simulink model "model1"  (R2024a)
settings: Solver=VariableStepAuto  StartTime=0.0  StopTime=simulation_time  RelTol=1e-3
values from neighbouring files (symbols this model uses):
  dq_0 = zeros(n, 1)    [example.m]
  path = @(t) circle_center + u_circle_plane*radius*cos((t/T) * (2*pi)) + v_circle_plane*radius*sin((t/T) * (2*pi))    [example.m]
  path_ddot = @(t) -u_circle_plane*radius*(2*pi/T)*(2*pi/T)*cos((t/T) * (2*pi)) - v_circle_plane*radius*(2*pi/T)*(2*pi/T)*sin((t/T) * (2*pi))    [example.m]
  path_dot = @(t) -u_circle_plane*radius*(2*pi/T)*sin((t/T) * (2*pi)) + v_circle_plane*radius*(2*pi/T)*cos((t/T) * (2*pi))    [example.m]
  q_0 = randn(n, 1)    [example.m]
  robot_model = importrobot("../robot_model/kuka-lwr-4plus/model1.urdf", 'DataFormat', 'column')    [example.m]
undefined symbols (not defined in the file or in its folder): torque_low_bound, torque_up_bound, X, Y, Z
libraries: sm_lib x74, nesl_utility x8, robotmaniplib x4
(part 2 of 5)

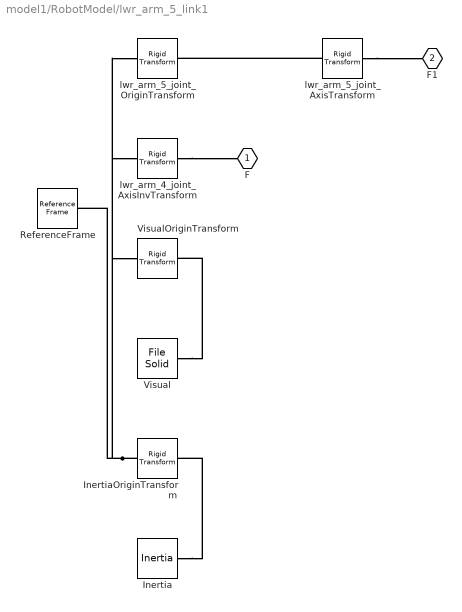
== system model1/RobotModel/lwr_arm_5_link1 ==
  Inertia : sm_lib/Body Elements/Inertia  InertiaType=Custom  Mass=2  MassUnits=kg  CenterOfMass=[0, 0, 0]  CenterOfMassUnits=m  MomentsOfInertia=[0.0126506666667, 0.0108506666667, 0.003]  MomentsOfInertiaUnits=kg*m^2  ProductsOfInertia=[0, 0, 0]  ProductsOfInertiaUnits=kg*m^2  GraphicType=None  MarkerShape=Inertia  MarkerSize=20  GraphicVisPropType=SimpleVisualProperties  GraphicDiffuseColor=[0.5 0.5 0.5]  GraphicOpacity=1  GraphicSpecularColor=[0.5 0.5 0.5 1.0]  GraphicAmbientColor=[0.15 0.15 0.15 1.0]  GraphicEmissiveColor=[0.0 0.0 0.0 1.0]  GraphicShininess=75
  InertiaOriginTransform : sm_lib/Frames and Transforms/Rigid Transform  RotationMethod=RotationSequence  FollAlignAxisA=+X  BaseAlignAxisA=+Y  FollAlignAxisB=+Y  BaseAlignAxisB=+Z  RotationStandardAxis=+Z  RotationAngle=0  RotationAngleUnits=deg  RotationArbitraryAxis=[0 0 1]  RotationSequenceAxes=BaseAxes  RotationSequence=XYZ  RotationSequenceAngles=[0, 0, 0]  RotationSequenceAnglesUnits=rad  RotationMatrix=[1 0 0;0 1 0;0 0 1]  Quaternion=[1 0 0 0]  TranslationMethod=Cartesian  TranslationCartesianOffset=[0, 0, 0.124]  TranslationCartesianOffsetUnits=m  TranslationStandardAxis=+Z  TranslationStandardOffset=0  TranslationStandardOffsetUnits=m  TranslationROffset=0  TranslationROffsetUnits=m  TranslationThetaOffset=0  TranslationThetaOffsetUnits=deg  TranslationZOffset=0  TranslationZOffsetUnits=m
  ReferenceFrame : sm_lib/Frames and Transforms/Reference Frame
  Visual : sm_lib/Body Elements/File Solid  ExtGeomFileName=/Users/salvatore/Desktop/Università/Development/Rob-HW/Damping-in-the-null-space-for-a-redundant-robot/robot_model/kuka-lwr-4plus/meshes/arm_segment_last.stl  UnitType=Custom  ExtGeomFileUnits=m  StepReaderType=HEX  ExportConvexHullGeometry=off  InertiaType=Custom  BasedOnType=DensityFromFile  Density=1000  DensityUnits=kg/m^3  Mass=0  MassUnits=kg  CenterOfMass=[0, 0, 0]  CenterOfMassUnits=m  MomentsOfInertia=[0, 0, 0]  MomentsOfInertiaUnits=kg*m^2  ProductsOfInertia=[0, 0, 0]  ProductsOfInertiaUnits=kg*m^2  GraphicType=FromGeometry  MarkerShape=Sphere  MarkerSize=10  GraphicVisPropType=SimpleVisualProperties  GraphicDiffuseColor=[1, 0.487, 0]  GraphicOpacity=1  GraphicSpecularColor=[0.5 0.5 0.5 1.0]  GraphicAmbientColor=[0.15 0.15 0.15 1.0]  GraphicEmissiveColor=[0.0 0.0 0.0 1.0]  GraphicShininess=75  DoExposeReferenceFrame=on  SerializedFrames=<Frames/>
  VisualOriginTransform : sm_lib/Frames and Transforms/Rigid Transform  RotationMethod=RotationSequence  FollAlignAxisA=+X  BaseAlignAxisA=+Y  FollAlignAxisB=+Y  BaseAlignAxisB=+Z  RotationStandardAxis=+Z  RotationAngle=0  RotationAngleUnits=deg  RotationArbitraryAxis=[0 0 1]  RotationSequenceAxes=BaseAxes  RotationSequence=XYZ  RotationSequenceAngles=[0, 0, -3.141592653589587]  RotationSequenceAnglesUnits=rad  RotationMatrix=[1 0 0;0 1 0;0 0 1]  Quaternion=[1 0 0 0]  TranslationMethod=Cartesian  TranslationCartesianOffset=[0, 0, 0]  TranslationCartesianOffsetUnits=m  TranslationStandardAxis=+Z  TranslationStandardOffset=0  TranslationStandardOffsetUnits=m  TranslationROffset=0  TranslationROffsetUnits=m  TranslationThetaOffset=0  TranslationThetaOffsetUnits=deg  TranslationZOffset=0  TranslationZOffsetUnits=m
  lwr_arm_4_joint_AxisInvTransform : sm_lib/Frames and Transforms/Rigid Transform  RotationMethod=ArbitraryAxis  FollAlignAxisA=+X  BaseAlignAxisA=+Y  FollAlignAxisB=+Y  BaseAlignAxisB=+Z  RotationStandardAxis=+Z  RotationAngle=0  RotationAngleUnits=rad  RotationArbitraryAxis=[1, 0, 0]  RotationSequenceAxes=FollowerAxes  RotationSequence=XYX  RotationSequenceAngles=[0 0 0]  RotationSequenceAnglesUnits=deg  RotationMatrix=[1 0 0;0 1 0;0 0 1]  Quaternion=[1 0 0 0]  TranslationMethod=Cartesian  TranslationCartesianOffset=[0, 0, 0]  TranslationCartesianOffsetUnits=m  TranslationStandardAxis=+Z  TranslationStandardOffset=0  TranslationStandardOffsetUnits=m  TranslationROffset=0  TranslationROffsetUnits=m  TranslationThetaOffset=0  TranslationThetaOffsetUnits=deg  TranslationZOffset=0  TranslationZOffsetUnits=m
  lwr_arm_5_joint_AxisTransform : sm_lib/Frames and Transforms/Rigid Transform  RotationMethod=ArbitraryAxis  FollAlignAxisA=+X  BaseAlignAxisA=+Y  FollAlignAxisB=+Y  BaseAlignAxisB=+Z  RotationStandardAxis=+Z  RotationAngle=1.570796326794897  RotationAngleUnits=rad  RotationArbitraryAxis=[1, 0, 0]  RotationSequenceAxes=FollowerAxes  RotationSequence=XYX  RotationSequenceAngles=[0 0 0]  RotationSequenceAnglesUnits=deg  RotationMatrix=[1 0 0;0 1 0;0 0 1]  Quaternion=[1 0 0 0]  TranslationMethod=Cartesian  TranslationCartesianOffset=[0, 0, 0]  TranslationCartesianOffsetUnits=m  TranslationStandardAxis=+Z  TranslationStandardOffset=0  TranslationStandardOffsetUnits=m  TranslationROffset=0  TranslationROffsetUnits=m  TranslationThetaOffset=0  TranslationThetaOffsetUnits=deg  TranslationZOffset=0  TranslationZOffsetUnits=m
  lwr_arm_5_joint_OriginTransform : sm_lib/Frames and Transforms/Rigid Transform  RotationMethod=RotationSequence  FollAlignAxisA=+X  BaseAlignAxisA=+Y  FollAlignAxisB=+Y  BaseAlignAxisB=+Z  RotationStandardAxis=+Z  RotationAngle=0  RotationAngleUnits=deg  RotationArbitraryAxis=[0 0 1]  RotationSequenceAxes=BaseAxes  RotationSequence=XYZ  RotationSequenceAngles=[0, 0, 0]  RotationSequenceAnglesUnits=rad  RotationMatrix=[1 0 0;0 1 0;0 0 1]  Quaternion=[1 0 0 0]  TranslationMethod=Cartesian  TranslationCartesianOffset=[0, 0, 0.19]  TranslationCartesianOffsetUnits=m  TranslationStandardAxis=+Z  TranslationStandardOffset=0  TranslationStandardOffsetUnits=m  TranslationROffset=0  TranslationROffsetUnits=m  TranslationThetaOffset=0  TranslationThetaOffsetUnits=deg  TranslationZOffset=0  TranslationZOffsetUnits=m
  F : PMIOPort  Side=Left
  F1 : PMIOPort  Port=2  Side=Right
  connections:
  Inertia/RConn1 -- InertiaOriginTransform/RConn1
  InertiaOriginTransform/LConn1 -- ReferenceFrame/RConn1 -- VisualOriginTransform/LConn1 -- lwr_arm_4_joint_AxisInvTransform/LConn1 -- lwr_arm_5_joint_OriginTransform/LConn1
  Visual/RConn1 -- VisualOriginTransform/RConn1
  lwr_arm_4_joint_AxisInvTransform/RConn1 -- F/RConn1
  lwr_arm_5_joint_AxisTransform/RConn1 -- F1/RConn1
  lwr_arm_5_joint_AxisTransform/LConn1 -- lwr_arm_5_joint_OriginTransform/RConn1

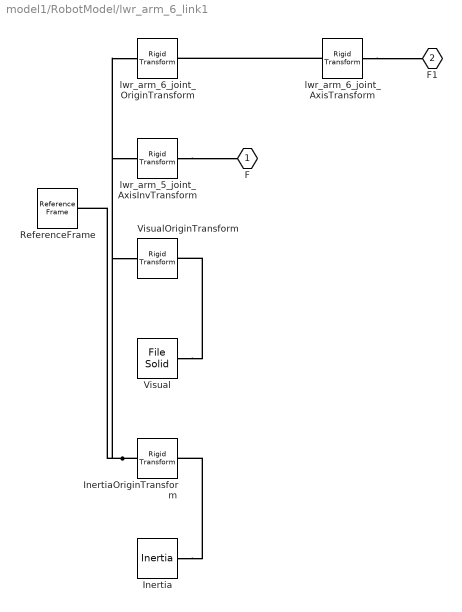
== system model1/RobotModel/lwr_arm_6_link1 ==
  Inertia : sm_lib/Body Elements/Inertia  InertiaType=Custom  Mass=1  MassUnits=kg  CenterOfMass=[0, 0, 0]  CenterOfMassUnits=m  MomentsOfInertia=[0.00260416666667, 0.00260416666667, 0.00260416666667]  MomentsOfInertiaUnits=kg*m^2  ProductsOfInertia=[0, 0, 0]  ProductsOfInertiaUnits=kg*m^2  GraphicType=None  MarkerShape=Inertia  MarkerSize=20  GraphicVisPropType=SimpleVisualProperties  GraphicDiffuseColor=[0.5 0.5 0.5]  GraphicOpacity=1  GraphicSpecularColor=[0.5 0.5 0.5 1.0]  GraphicAmbientColor=[0.15 0.15 0.15 1.0]  GraphicEmissiveColor=[0.0 0.0 0.0 1.0]  GraphicShininess=75
  InertiaOriginTransform : sm_lib/Frames and Transforms/Rigid Transform  RotationMethod=RotationSequence  FollAlignAxisA=+X  BaseAlignAxisA=+Y  FollAlignAxisB=+Y  BaseAlignAxisB=+Z  RotationStandardAxis=+Z  RotationAngle=0  RotationAngleUnits=deg  RotationArbitraryAxis=[0 0 1]  RotationSequenceAxes=BaseAxes  RotationSequence=XYZ  RotationSequenceAngles=[0, 0, 0]  RotationSequenceAnglesUnits=rad  RotationMatrix=[1 0 0;0 1 0;0 0 1]  Quaternion=[1 0 0 0]  TranslationMethod=Cartesian  TranslationCartesianOffset=[0, 0, 0]  TranslationCartesianOffsetUnits=m  TranslationStandardAxis=+Z  TranslationStandardOffset=0  TranslationStandardOffsetUnits=m  TranslationROffset=0  TranslationROffsetUnits=m  TranslationThetaOffset=0  TranslationThetaOffsetUnits=deg  TranslationZOffset=0  TranslationZOffsetUnits=m
  ReferenceFrame : sm_lib/Frames and Transforms/Reference Frame
  Visual : sm_lib/Body Elements/File Solid  ExtGeomFileName=/Users/salvatore/Desktop/Università/Development/Rob-HW/Damping-in-the-null-space-for-a-redundant-robot/robot_model/kuka-lwr-4plus/meshes/arm_wrist.stl  UnitType=Custom  ExtGeomFileUnits=m  StepReaderType=HEX  ExportConvexHullGeometry=off  InertiaType=Custom  BasedOnType=DensityFromFile  Density=1000  DensityUnits=kg/m^3  Mass=0  MassUnits=kg  CenterOfMass=[0, 0, 0]  CenterOfMassUnits=m  MomentsOfInertia=[0, 0, 0]  MomentsOfInertiaUnits=kg*m^2  ProductsOfInertia=[0, 0, 0]  ProductsOfInertiaUnits=kg*m^2  GraphicType=FromGeometry  MarkerShape=Sphere  MarkerSize=10  GraphicVisPropType=SimpleVisualProperties  GraphicDiffuseColor=[0.7, 0.7, 0.7]  GraphicOpacity=1  GraphicSpecularColor=[0.5 0.5 0.5 1.0]  GraphicAmbientColor=[0.15 0.15 0.15 1.0]  GraphicEmissiveColor=[0.0 0.0 0.0 1.0]  GraphicShininess=75  DoExposeReferenceFrame=on  SerializedFrames=<Frames/>
  VisualOriginTransform : sm_lib/Frames and Transforms/Rigid Transform  RotationMethod=RotationSequence  FollAlignAxisA=+X  BaseAlignAxisA=+Y  FollAlignAxisB=+Y  BaseAlignAxisB=+Z  RotationStandardAxis=+Z  RotationAngle=0  RotationAngleUnits=deg  RotationArbitraryAxis=[0 0 1]  RotationSequenceAxes=BaseAxes  RotationSequence=XYZ  RotationSequenceAngles=[0, 0, -3.141592653589587]  RotationSequenceAnglesUnits=rad  RotationMatrix=[1 0 0;0 1 0;0 0 1]  Quaternion=[1 0 0 0]  TranslationMethod=Cartesian  TranslationCartesianOffset=[0, 0, 0]  TranslationCartesianOffsetUnits=m  TranslationStandardAxis=+Z  TranslationStandardOffset=0  TranslationStandardOffsetUnits=m  TranslationROffset=0  TranslationROffsetUnits=m  TranslationThetaOffset=0  TranslationThetaOffsetUnits=deg  TranslationZOffset=0  TranslationZOffsetUnits=m
  lwr_arm_5_joint_AxisInvTransform : sm_lib/Frames and Transforms/Rigid Transform  RotationMethod=ArbitraryAxis  FollAlignAxisA=+X  BaseAlignAxisA=+Y  FollAlignAxisB=+Y  BaseAlignAxisB=+Z  RotationStandardAxis=+Z  RotationAngle=1.570796326794897  RotationAngleUnits=rad  RotationArbitraryAxis=[1, 0, 0]  RotationSequenceAxes=FollowerAxes  RotationSequence=XYX  RotationSequenceAngles=[0 0 0]  RotationSequenceAnglesUnits=deg  RotationMatrix=[1 0 0;0 1 0;0 0 1]  Quaternion=[1 0 0 0]  TranslationMethod=Cartesian  TranslationCartesianOffset=[0, 0, 0]  TranslationCartesianOffsetUnits=m  TranslationStandardAxis=+Z  TranslationStandardOffset=0  TranslationStandardOffsetUnits=m  TranslationROffset=0  TranslationROffsetUnits=m  TranslationThetaOffset=0  TranslationThetaOffsetUnits=deg  TranslationZOffset=0  TranslationZOffsetUnits=m
  lwr_arm_6_joint_AxisTransform : sm_lib/Frames and Transforms/Rigid Transform  RotationMethod=ArbitraryAxis  FollAlignAxisA=+X  BaseAlignAxisA=+Y  FollAlignAxisB=+Y  BaseAlignAxisB=+Z  RotationStandardAxis=+Z  RotationAngle=0  RotationAngleUnits=rad  RotationArbitraryAxis=[1, 0, 0]  RotationSequenceAxes=FollowerAxes  RotationSequence=XYX  RotationSequenceAngles=[0 0 0]  RotationSequenceAnglesUnits=deg  RotationMatrix=[1 0 0;0 1 0;0 0 1]  Quaternion=[1 0 0 0]  TranslationMethod=Cartesian  TranslationCartesianOffset=[0, 0, 0]  TranslationCartesianOffsetUnits=m  TranslationStandardAxis=+Z  TranslationStandardOffset=0  TranslationStandardOffsetUnits=m  TranslationROffset=0  TranslationROffsetUnits=m  TranslationThetaOffset=0  TranslationThetaOffsetUnits=deg  TranslationZOffset=0  TranslationZOffsetUnits=m
  lwr_arm_6_joint_OriginTransform : sm_lib/Frames and Transforms/Rigid Transform  RotationMethod=RotationSequence  FollAlignAxisA=+X  BaseAlignAxisA=+Y  FollAlignAxisB=+Y  BaseAlignAxisB=+Z  RotationStandardAxis=+Z  RotationAngle=0  RotationAngleUnits=deg  RotationArbitraryAxis=[0 0 1]  RotationSequenceAxes=BaseAxes  RotationSequence=XYZ  RotationSequenceAngles=[0, -0, 0]  RotationSequenceAnglesUnits=rad  RotationMatrix=[1 0 0;0 1 0;0 0 1]  Quaternion=[1 0 0 0]  TranslationMethod=Cartesian  TranslationCartesianOffset=[0, 0, 0]  TranslationCartesianOffsetUnits=m  TranslationStandardAxis=+Z  TranslationStandardOffset=0  TranslationStandardOffsetUnits=m  TranslationROffset=0  TranslationROffsetUnits=m  TranslationThetaOffset=0  TranslationThetaOffsetUnits=deg  TranslationZOffset=0  TranslationZOffsetUnits=m
  F : PMIOPort  Side=Left
  F1 : PMIOPort  Port=2  Side=Right
  connections:
  Inertia/RConn1 -- InertiaOriginTransform/RConn1
  InertiaOriginTransform/LConn1 -- ReferenceFrame/RConn1 -- VisualOriginTransform/LConn1 -- lwr_arm_5_joint_AxisInvTransform/LConn1 -- lwr_arm_6_joint_OriginTransform/LConn1
  Visual/RConn1 -- VisualOriginTransform/RConn1
  lwr_arm_5_joint_AxisInvTransform/RConn1 -- F/RConn1
  lwr_arm_6_joint_AxisTransform/RConn1 -- F1/RConn1
  lwr_arm_6_joint_AxisTransform/LConn1 -- lwr_arm_6_joint_OriginTransform/RConn1

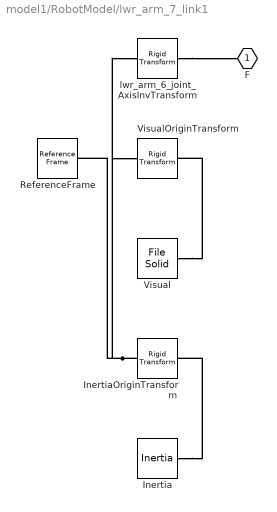
== system model1/RobotModel/lwr_arm_7_link1 ==
  Inertia : sm_lib/Body Elements/Inertia  InertiaType=Custom  Mass=0.2  MassUnits=kg  CenterOfMass=[0, 0, 0]  CenterOfMassUnits=m  MomentsOfInertia=[6.66666666667e-05, 6.66666666667e-05, 0.00012]  MomentsOfInertiaUnits=kg*m^2  ProductsOfInertia=[0, 0, 0]  ProductsOfInertiaUnits=kg*m^2  GraphicType=None  MarkerShape=Inertia  MarkerSize=20  GraphicVisPropType=SimpleVisualProperties  GraphicDiffuseColor=[0.5 0.5 0.5]  GraphicOpacity=1  GraphicSpecularColor=[0.5 0.5 0.5 1.0]  GraphicAmbientColor=[0.15 0.15 0.15 1.0]  GraphicEmissiveColor=[0.0 0.0 0.0 1.0]  GraphicShininess=75
  InertiaOriginTransform : sm_lib/Frames and Transforms/Rigid Transform  RotationMethod=RotationSequence  FollAlignAxisA=+X  BaseAlignAxisA=+Y  FollAlignAxisB=+Y  BaseAlignAxisB=+Z  RotationStandardAxis=+Z  RotationAngle=0  RotationAngleUnits=deg  RotationArbitraryAxis=[0 0 1]  RotationSequenceAxes=BaseAxes  RotationSequence=XYZ  RotationSequenceAngles=[0, 0, 0]  RotationSequenceAnglesUnits=rad  RotationMatrix=[1 0 0;0 1 0;0 0 1]  Quaternion=[1 0 0 0]  TranslationMethod=Cartesian  TranslationCartesianOffset=[0, 0, 0]  TranslationCartesianOffsetUnits=m  TranslationStandardAxis=+Z  TranslationStandardOffset=0  TranslationStandardOffsetUnits=m  TranslationROffset=0  TranslationROffsetUnits=m  TranslationThetaOffset=0  TranslationThetaOffsetUnits=deg  TranslationZOffset=0  TranslationZOffsetUnits=m
  ReferenceFrame : sm_lib/Frames and Transforms/Reference Frame
  Visual : sm_lib/Body Elements/File Solid  ExtGeomFileName=/Users/salvatore/Desktop/Università/Development/Rob-HW/Damping-in-the-null-space-for-a-redundant-robot/robot_model/kuka-lwr-4plus/meshes/arm_flanche.stl  UnitType=Custom  ExtGeomFileUnits=m  StepReaderType=HEX  ExportConvexHullGeometry=off  InertiaType=Custom  BasedOnType=DensityFromFile  Density=1000  DensityUnits=kg/m^3  Mass=0  MassUnits=kg  CenterOfMass=[0, 0, 0]  CenterOfMassUnits=m  MomentsOfInertia=[0, 0, 0]  MomentsOfInertiaUnits=kg*m^2  ProductsOfInertia=[0, 0, 0]  ProductsOfInertiaUnits=kg*m^2  GraphicType=FromGeometry  MarkerShape=Sphere  MarkerSize=10  GraphicVisPropType=SimpleVisualProperties  GraphicDiffuseColor=[0.7, 0.7, 0.7]  GraphicOpacity=1  GraphicSpecularColor=[0.5 0.5 0.5 1.0]  GraphicAmbientColor=[0.15 0.15 0.15 1.0]  GraphicEmissiveColor=[0.0 0.0 0.0 1.0]  GraphicShininess=75  DoExposeReferenceFrame=on  SerializedFrames=<Frames/>
  VisualOriginTransform : sm_lib/Frames and Transforms/Rigid Transform  RotationMethod=RotationSequence  FollAlignAxisA=+X  BaseAlignAxisA=+Y  FollAlignAxisB=+Y  BaseAlignAxisB=+Z  RotationStandardAxis=+Z  RotationAngle=0  RotationAngleUnits=deg  RotationArbitraryAxis=[0 0 1]  RotationSequenceAxes=BaseAxes  RotationSequence=XYZ  RotationSequenceAngles=[0, 0, 0]  RotationSequenceAnglesUnits=rad  RotationMatrix=[1 0 0;0 1 0;0 0 1]  Quaternion=[1 0 0 0]  TranslationMethod=Cartesian  TranslationCartesianOffset=[0, 0, 0]  TranslationCartesianOffsetUnits=m  TranslationStandardAxis=+Z  TranslationStandardOffset=0  TranslationStandardOffsetUnits=m  TranslationROffset=0  TranslationROffsetUnits=m  TranslationThetaOffset=0  TranslationThetaOffsetUnits=deg  TranslationZOffset=0  TranslationZOffsetUnits=m
  lwr_arm_6_joint_AxisInvTransform : sm_lib/Frames and Transforms/Rigid Transform  RotationMethod=ArbitraryAxis  FollAlignAxisA=+X  BaseAlignAxisA=+Y  FollAlignAxisB=+Y  BaseAlignAxisB=+Z  RotationStandardAxis=+Z  RotationAngle=0  RotationAngleUnits=rad  RotationArbitraryAxis=[1, 0, 0]  RotationSequenceAxes=FollowerAxes  RotationSequence=XYX  RotationSequenceAngles=[0 0 0]  RotationSequenceAnglesUnits=deg  RotationMatrix=[1 0 0;0 1 0;0 0 1]  Quaternion=[1 0 0 0]  TranslationMethod=Cartesian  TranslationCartesianOffset=[0, 0, 0]  TranslationCartesianOffsetUnits=m  TranslationStandardAxis=+Z  TranslationStandardOffset=0  TranslationStandardOffsetUnits=m  TranslationROffset=0  TranslationROffsetUnits=m  TranslationThetaOffset=0  TranslationThetaOffsetUnits=deg  TranslationZOffset=0  TranslationZOffsetUnits=m
  F : PMIOPort  Side=Left
  connections:
  Inertia/RConn1 -- InertiaOriginTransform/RConn1
  InertiaOriginTransform/LConn1 -- ReferenceFrame/RConn1 -- VisualOriginTransform/LConn1 -- lwr_arm_6_joint_AxisInvTransform/LConn1
  Visual/RConn1 -- VisualOriginTransform/RConn1
  lwr_arm_6_joint_AxisInvTransform/RConn1 -- F/RConn1

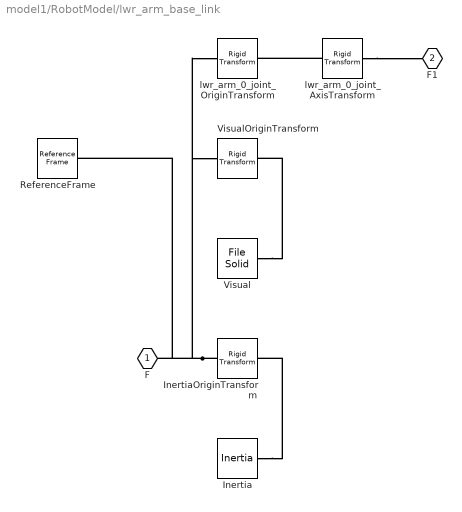
== system model1/RobotModel/lwr_arm_base_link ==
  Inertia : sm_lib/Body Elements/Inertia  InertiaType=Custom  Mass=1.2  MassUnits=kg  CenterOfMass=[0, 0, 0]  CenterOfMassUnits=m  MomentsOfInertia=[0.00229, 0.00216, 0.00229]  MomentsOfInertiaUnits=kg*m^2  ProductsOfInertia=[0, 0, 0]  ProductsOfInertiaUnits=kg*m^2  GraphicType=None  MarkerShape=Inertia  MarkerSize=20  GraphicVisPropType=SimpleVisualProperties  GraphicDiffuseColor=[0.5 0.5 0.5]  GraphicOpacity=1  GraphicSpecularColor=[0.5 0.5 0.5 1.0]  GraphicAmbientColor=[0.15 0.15 0.15 1.0]  GraphicEmissiveColor=[0.0 0.0 0.0 1.0]  GraphicShininess=75
  InertiaOriginTransform : sm_lib/Frames and Transforms/Rigid Transform  RotationMethod=RotationSequence  FollAlignAxisA=+X  BaseAlignAxisA=+Y  FollAlignAxisB=+Y  BaseAlignAxisB=+Z  RotationStandardAxis=+Z  RotationAngle=0  RotationAngleUnits=deg  RotationArbitraryAxis=[0 0 1]  RotationSequenceAxes=BaseAxes  RotationSequence=XYZ  RotationSequenceAngles=[0, 0, 0]  RotationSequenceAnglesUnits=rad  RotationMatrix=[1 0 0;0 1 0;0 0 1]  Quaternion=[1 0 0 0]  TranslationMethod=Cartesian  TranslationCartesianOffset=[0, 0, 0.055]  TranslationCartesianOffsetUnits=m  TranslationStandardAxis=+Z  TranslationStandardOffset=0  TranslationStandardOffsetUnits=m  TranslationROffset=0  TranslationROffsetUnits=m  TranslationThetaOffset=0  TranslationThetaOffsetUnits=deg  TranslationZOffset=0  TranslationZOffsetUnits=m
  ReferenceFrame : sm_lib/Frames and Transforms/Reference Frame
  Visual : sm_lib/Body Elements/File Solid  ExtGeomFileName=/Users/salvatore/Desktop/Università/Development/Rob-HW/Damping-in-the-null-space-for-a-redundant-robot/robot_model/kuka-lwr-4plus/meshes/arm_base.stl  UnitType=Custom  ExtGeomFileUnits=m  StepReaderType=HEX  ExportConvexHullGeometry=off  InertiaType=Custom  BasedOnType=DensityFromFile  Density=1000  DensityUnits=kg/m^3  Mass=0  MassUnits=kg  CenterOfMass=[0, 0, 0]  CenterOfMassUnits=m  MomentsOfInertia=[0, 0, 0]  MomentsOfInertiaUnits=kg*m^2  ProductsOfInertia=[0, 0, 0]  ProductsOfInertiaUnits=kg*m^2  GraphicType=FromGeometry  MarkerShape=Sphere  MarkerSize=10  GraphicVisPropType=SimpleVisualProperties  GraphicDiffuseColor=[1, 0.487, 0]  GraphicOpacity=1  GraphicSpecularColor=[0.5 0.5 0.5 1.0]  GraphicAmbientColor=[0.15 0.15 0.15 1.0]  GraphicEmissiveColor=[0.0 0.0 0.0 1.0]  GraphicShininess=75  DoExposeReferenceFrame=on  SerializedFrames=<Frames/>
  VisualOriginTransform : sm_lib/Frames and Transforms/Rigid Transform  RotationMethod=RotationSequence  FollAlignAxisA=+X  BaseAlignAxisA=+Y  FollAlignAxisB=+Y  BaseAlignAxisB=+Z  RotationStandardAxis=+Z  RotationAngle=0  RotationAngleUnits=deg  RotationArbitraryAxis=[0 0 1]  RotationSequenceAxes=BaseAxes  RotationSequence=XYZ  RotationSequenceAngles=[0, 0, 0]  RotationSequenceAnglesUnits=rad  RotationMatrix=[1 0 0;0 1 0;0 0 1]  Quaternion=[1 0 0 0]  TranslationMethod=Cartesian  TranslationCartesianOffset=[0, 0, 0]  TranslationCartesianOffsetUnits=m  TranslationStandardAxis=+Z  TranslationStandardOffset=0  TranslationStandardOffsetUnits=m  TranslationROffset=0  TranslationROffsetUnits=m  TranslationThetaOffset=0  TranslationThetaOffsetUnits=deg  TranslationZOffset=0  TranslationZOffsetUnits=m
  lwr_arm_0_joint_AxisTransform : sm_lib/Frames and Transforms/Rigid Transform  RotationMethod=ArbitraryAxis  FollAlignAxisA=+X  BaseAlignAxisA=+Y  FollAlignAxisB=+Y  BaseAlignAxisB=+Z  RotationStandardAxis=+Z  RotationAngle=0  RotationAngleUnits=rad  RotationArbitraryAxis=[1, 0, 0]  RotationSequenceAxes=FollowerAxes  RotationSequence=XYX  RotationSequenceAngles=[0 0 0]  RotationSequenceAnglesUnits=deg  RotationMatrix=[1 0 0;0 1 0;0 0 1]  Quaternion=[1 0 0 0]  TranslationMethod=Cartesian  TranslationCartesianOffset=[0, 0, 0]  TranslationCartesianOffsetUnits=m  TranslationStandardAxis=+Z  TranslationStandardOffset=0  TranslationStandardOffsetUnits=m  TranslationROffset=0  TranslationROffsetUnits=m  TranslationThetaOffset=0  TranslationThetaOffsetUnits=deg  TranslationZOffset=0  TranslationZOffsetUnits=m
  lwr_arm_0_joint_OriginTransform : sm_lib/Frames and Transforms/Rigid Transform  RotationMethod=RotationSequence  FollAlignAxisA=+X  BaseAlignAxisA=+Y  FollAlignAxisB=+Y  BaseAlignAxisB=+Z  RotationStandardAxis=+Z  RotationAngle=0  RotationAngleUnits=deg  RotationArbitraryAxis=[0 0 1]  RotationSequenceAxes=BaseAxes  RotationSequence=XYZ  RotationSequenceAngles=[0, 0, 0]  RotationSequenceAnglesUnits=rad  RotationMatrix=[1 0 0;0 1 0;0 0 1]  Quaternion=[1 0 0 0]  TranslationMethod=Cartesian  TranslationCartesianOffset=[0, 0, 0.11]  TranslationCartesianOffsetUnits=m  TranslationStandardAxis=+Z  TranslationStandardOffset=0  TranslationStandardOffsetUnits=m  TranslationROffset=0  TranslationROffsetUnits=m  TranslationThetaOffset=0  TranslationThetaOffsetUnits=deg  TranslationZOffset=0  TranslationZOffsetUnits=m
  F : PMIOPort  Side=Left
  F1 : PMIOPort  Port=2  Side=Right
  connections:
  Inertia/RConn1 -- InertiaOriginTransform/RConn1
  ReferenceFrame/RConn1 -- InertiaOriginTransform/LConn1 -- VisualOriginTransform/LConn1 -- lwr_arm_0_joint_OriginTransform/LConn1 -- F/RConn1
  Visual/RConn1 -- VisualOriginTransform/RConn1
  lwr_arm_0_joint_AxisTransform/RConn1 -- F1/RConn1
  lwr_arm_0_joint_AxisTransform/LConn1 -- lwr_arm_0_joint_OriginTransform/RConn1

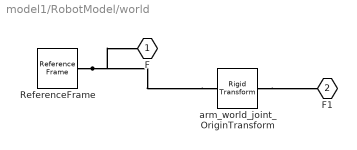
== system model1/RobotModel/world ==
  ReferenceFrame : sm_lib/Frames and Transforms/Reference Frame
  arm_world_joint_OriginTransform : sm_lib/Frames and Transforms/Rigid Transform  RotationMethod=RotationSequence  FollAlignAxisA=+X  BaseAlignAxisA=+Y  FollAlignAxisB=+Y  BaseAlignAxisB=+Z  RotationStandardAxis=+Z  RotationAngle=0  RotationAngleUnits=deg  RotationArbitraryAxis=[0 0 1]  RotationSequenceAxes=BaseAxes  RotationSequence=XYZ  RotationSequenceAngles=[0, 0, 0]  RotationSequenceAnglesUnits=rad  RotationMatrix=[1 0 0;0 1 0;0 0 1]  Quaternion=[1 0 0 0]  TranslationMethod=Cartesian  TranslationCartesianOffset=[0, 0, 0.01]  TranslationCartesianOffsetUnits=m  TranslationStandardAxis=+Z  TranslationStandardOffset=0  TranslationStandardOffsetUnits=m  TranslationROffset=0  TranslationROffsetUnits=m  TranslationThetaOffset=0  TranslationThetaOffsetUnits=deg  TranslationZOffset=0  TranslationZOffsetUnits=m
  F : PMIOPort  Side=Left
  F1 : PMIOPort  Port=2  Side=Right
  connections:
  arm_world_joint_OriginTransform/LConn1 -- ReferenceFrame/RConn1 -- F/RConn1
  arm_world_joint_OriginTransform/RConn1 -- F1/RConn1

== matlab function model1/MATLAB Function ==
  data: configuration input; g_num output
function g_num = g_num(configuration)
%G_NUM1
%    G_NUM = G_NUM1(Q1,Q2,Q3,Q4,Q5)

%    This function was generated by the Symbolic Math Toolbox version 24.1.
%    01-Jul-2024 12:17:42

q1 = configuration(1);
q2 = configuration(2);
q3 = configuration(3);
q4 = configuration(4);
q5 = configuration(5);

t2 = cos(q1);
t3 = cos(q2);
t4 = cos(q3);
t5 = cos(q4);
t6 = cos(q5);
t7 = sin(q1);
t8 = sin(q2);
t9 = sin(q3);
t10 = sin(q4);
t11 = sin(q5);
t12 = t2.*t4;
t13 = t2.*t9;
t14 = t3.*t4.*t7;
t15 = t3.*t7.*t9;
t16 = -t15;
t17 = t13+t14;
t18 = t12+t16;
mt1 = [t7.*(9.31e+2./2.5e+2)-t2.*t8.*3.0772e+1-t4.*t7.*(9.31e+2./2.5e+2)-t3.*t13.*(9.31e+2./2.5e+2)-t2.*t5.*t8.*1.36024e+1+t4.*t6.*t7.*2.4304+t3.*t6.*t13.*2.4304+t3.*t10.*t12.*1.36024e+1-t7.*t9.*t10.*1.36024e+1+t2.*t8.*t10.*t11.*2.4304+t3.*t5.*t11.*t12.*2.4304-t5.*t7.*t9.*t11.*2.4304];
mt2 = [t7.*(t3.*3.14e+2+t3.*t5.*(6.94e+2./5.0)-t8.*t9.*3.8e+1+t4.*t8.*t10.*(6.94e+2./5.0)+t6.*t8.*t9.*(1.24e+2./5.0)-t3.*t10.*t11.*(1.24e+2./5.0)+t4.*t5.*t8.*t11.*(1.24e+2./5.0)).*(-4.9e+1./5.0e+2);t13.*(-9.31e+2./2.5e+2)-t14.*(9.31e+2./2.5e+2)+t6.*t17.*2.4304+t10.*t18.*1.36024e+1+t5.*t11.*t18.*2.4304;t11.*(t10.*t17-t5.*t7.*t8).*(-2.4304)+t5.*t17.*1.36024e+1+t7.*t8.*t10.*1.36024e+1];
mt3 = [t6.*(t5.*t17+t7.*t8.*t10).*2.4304+t11.*t18.*2.4304;0.0;0.0];
g_num = [mt1;mt2;mt3];
end

== matlab function model1/Feeback linearization acceleration ==
  data: f_q input; tau output; dq input; p_d input; dp_d input; ddp_d input; j input; g_q input; c input; M input; jdot input
function tau = FBLAcceleration(f_q, dq, p_d, dp_d, ddp_d, j, g_q, c, M, jdot)

% Control gains
K_P = 100;
K_D = 10;

K_V = 10;
K_M = 10;

% Acceleration command of the FBL controller
% a   = ddq_d + K_P*(q_d - q) + K_D*(dq_d - dq);

% tau = j' * K_P * (p_d - f_q) + K_D * (pinv(j)*dp_d - dq) + g_q;
% end

Winv = M; % the inverse of the weight matrix: can be inverse of eye(7), m^-1, m^-2 
% F = j * pinv(M);
% Finv = pinv(F);
F = j / M; % equivalent to j * inv(M)
Finv = (Winv * F') / (F * Winv * F'); % the weighted pseudo-inverse of F = W^-1*F'*(F*W^-1*F')^-1
a = ddp_d + K_D*(dp_d - j*dq) + K_P*(p_d - f_q);
u0 = zeros(7,1);  % No null space term / no damping
% u0 = -K_V * dq;  % velocity damping
% u0 = -K_M * M * dq;  % momentum damping
tau = Finv * (a - jdot*dq + F*(c + g_q)) + (eye(7) - Finv*F)*u0;

end

== matlab function model1/MATLAB Function1 ==
  data: configuration input; j output
function j = analytic_jacobian(configuration)
%ANALYTIC_JACOBIAN1
%    J = ANALYTIC_JACOBIAN1(Q1,Q2,Q3,Q4)

%    This function was generated by the Symbolic Math Toolbox version 24.1.
%    02-Jul-2024 11:08:16

q1 = configuration(1);
q2 = configuration(2);
q3 = configuration(3);
q4 = configuration(4);

t2 = cos(q1);
t3 = cos(q2);
t4 = cos(q3);
t5 = cos(q4);
t6 = sin(q1);
t7 = sin(q2);
t8 = sin(q3);
t9 = sin(q4);
t10 = t2.*t8;
t11 = t6.*t8;
t12 = t2.*t3.*t4;
t13 = t3.*t4.*t6;
t14 = -t12;
t15 = t10+t13;
t16 = t11+t14;
mt1 = [t6.*t7.*(2.0./5.0)-t9.*t15.*(3.9e+1./1.0e+2)+t5.*t6.*t7.*(3.9e+1./1.0e+2),t2.*t7.*(-2.0./5.0)-t9.*t16.*(3.9e+1./1.0e+2)-t2.*t5.*t7.*(3.9e+1./1.0e+2),0.0,t2.*t3.*(-2.0./5.0)-t2.*t3.*t5.*(3.9e+1./1.0e+2)-t2.*t4.*t7.*t9.*(3.9e+1./1.0e+2),t3.*t6.*(-2.0./5.0)-t3.*t5.*t6.*(3.9e+1./1.0e+2)-t4.*t6.*t7.*t9.*(3.9e+1./1.0e+2),t7.*(-2.0./5.0)-t5.*t7.*(3.9e+1./1.0e+2)+t3.*t4.*t9.*(3.9e+1./1.0e+2),t9.*(t4.*t6+t3.*t10).*(-3.9e+1./1.0e+2),t9.*(t2.*t4-t3.*t11).*(3.9e+1./1.0e+2),t7.*t8.*t9.*(-3.9e+1./1.0e+2)];
mt2 = [t5.*t16.*(-3.9e+1./1.0e+2)+t2.*t7.*t9.*(3.9e+1./1.0e+2),t5.*t15.*(3.9e+1./1.0e+2)+t6.*t7.*t9.*(3.9e+1./1.0e+2),t3.*t9.*(-3.9e+1./1.0e+2)+t4.*t5.*t7.*(3.9e+1./1.0e+2),0.0,0.0,0.0,0.0,0.0,0.0,0.0,0.0,0.0];
j = reshape([mt1,mt2],3,7);
end

== matlab function model1/MATLAB Function3 ==
  data: currJointPos input; j_dot output; currJointVel input
function j_dot = analytic_j_dot1(currJointPos, currJointVel)
%ANALYTIC_J_DOT1
%    J_DOT = ANALYTIC_J_DOT1(Q1,Q2,Q3,Q4,Q_DOT1,Q_DOT2,Q_DOT3,Q_DOT4)

%    This function was generated by the Symbolic Math Toolbox version 24.1.
%    02-Jul-2024 11:08:30

q1 = currJointPos(1);
q_dot1 = currJointVel(1);
q2 = currJointPos(2);
q_dot2 = currJointVel(2);
q3 = currJointPos(3);
q_dot3 = currJointVel(3);
q4 = currJointPos(4);
q_dot4 = currJointVel(4);

t2 = cos(q1);
t3 = cos(q2);
t4 = cos(q3);
t5 = cos(q4);
t6 = sin(q1);
t7 = sin(q2);
t8 = sin(q3);
t9 = sin(q4);
t10 = t2.*t8;
t11 = t6.*t8;
t12 = q_dot3.*t2.*t4;
t14 = q_dot3.*t4.*t6;
t16 = t2.*t3.*t4;
t17 = t3.*t4.*t6;
t20 = q_dot2.*t2.*t4.*t7;
t22 = q_dot2.*t4.*t6.*t7;
t13 = q_dot1.*t10;
t15 = q_dot1.*t11;
t18 = q_dot1.*t16;
t19 = q_dot1.*t17;
t21 = q_dot3.*t3.*t10;
t23 = q_dot3.*t3.*t11;
t24 = -t12;
t25 = -t16;
t27 = t10+t17;
t26 = -t18;
t28 = t11+t25;
t29 = t13+t14+t19+t20+t21;
t30 = t15+t22+t23+t24+t26;
mt1 = [t9.*t30.*(3.9e+1./1.0e+2)+q_dot1.*t2.*t7.*(2.0./5.0)+q_dot2.*t3.*t6.*(2.0./5.0)-q_dot4.*t5.*t27.*(3.9e+1./1.0e+2)+q_dot1.*t2.*t5.*t7.*(3.9e+1./1.0e+2)+q_dot2.*t3.*t5.*t6.*(3.9e+1./1.0e+2)-q_dot4.*t6.*t7.*t9.*(3.9e+1./1.0e+2),t9.*t29.*(-3.9e+1./1.0e+2)-q_dot2.*t2.*t3.*(2.0./5.0)+q_dot1.*t6.*t7.*(2.0./5.0)-q_dot4.*t5.*t28.*(3.9e+1./1.0e+2)-q_dot2.*t2.*t3.*t5.*(3.9e+1./1.0e+2)+q_dot1.*t5.*t6.*t7.*(3.9e+1./1.0e+2)+q_dot4.*t2.*t7.*t9.*(3.9e+1./1.0e+2),0.0];
mt2 = [q_dot1.*t3.*t6.*(2.0./5.0)+q_dot2.*t2.*t7.*(2.0./5.0)-q_dot2.*t9.*t16.*(3.9e+1./1.0e+2)+q_dot1.*t3.*t5.*t6.*(3.9e+1./1.0e+2)+q_dot2.*t2.*t5.*t7.*(3.9e+1./1.0e+2)+q_dot4.*t2.*t3.*t9.*(3.9e+1./1.0e+2)+q_dot3.*t7.*t9.*t10.*(3.9e+1./1.0e+2)-q_dot4.*t2.*t4.*t5.*t7.*(3.9e+1./1.0e+2)+q_dot1.*t4.*t6.*t7.*t9.*(3.9e+1./1.0e+2),q_dot1.*t2.*t3.*(-2.0./5.0)+q_dot2.*t6.*t7.*(2.0./5.0)-q_dot2.*t9.*t17.*(3.9e+1./1.0e+2)-q_dot1.*t2.*t3.*t5.*(3.9e+1./1.0e+2)+q_dot2.*t5.*t6.*t7.*(3.9e+1./1.0e+2)+q_dot4.*t3.*t6.*t9.*(3.9e+1./1.0e+2)+q_dot3.*t7.*t9.*t11.*(3.9e+1./1.0e+2)-q_dot1.*t2.*t4.*t7.*t9.*(3.9e+1./1.0e+2)-q_dot4.*t4.*t5.*t6.*t7.*(3.9e+1./1.0e+2)];
mt3 = [q_dot2.*t3.*(-2.0./5.0)-q_dot2.*t3.*t5.*(3.9e+1./1.0e+2)+q_dot4.*t7.*t9.*(3.9e+1./1.0e+2)+q_dot4.*t3.*t4.*t5.*(3.9e+1./1.0e+2)-q_dot2.*t4.*t7.*t9.*(3.9e+1./1.0e+2)-q_dot3.*t3.*t8.*t9.*(3.9e+1./1.0e+2),t9.*(q_dot3.*t11+t3.*t15+t3.*t24-q_dot1.*t2.*t4+q_dot2.*t7.*t10).*(3.9e+1./1.0e+2)-q_dot4.*t5.*(t4.*t6+t3.*t10).*(3.9e+1./1.0e+2),t9.*(q_dot3.*t10+t3.*t13+t3.*t14+q_dot1.*t4.*t6-q_dot2.*t7.*t11).*(-3.9e+1./1.0e+2)+q_dot4.*t5.*(t2.*t4-t3.*t11).*(3.9e+1./1.0e+2),q_dot2.*t3.*t8.*t9.*(-3.9e+1./1.0e+2)-q_dot3.*t4.*t7.*t9.*(3.9e+1./1.0e+2)-q_dot4.*t5.*t7.*t8.*(3.9e+1./1.0e+2)];
mt4 = [t5.*t29.*(-3.9e+1./1.0e+2)+q_dot4.*t9.*t28.*(3.9e+1./1.0e+2)+q_dot2.*t2.*t3.*t9.*(3.9e+1./1.0e+2)+q_dot4.*t2.*t5.*t7.*(3.9e+1./1.0e+2)-q_dot1.*t6.*t7.*t9.*(3.9e+1./1.0e+2),t5.*t30.*(-3.9e+1./1.0e+2)-q_dot4.*t9.*t27.*(3.9e+1./1.0e+2)+q_dot1.*t2.*t7.*t9.*(3.9e+1./1.0e+2)+q_dot2.*t3.*t6.*t9.*(3.9e+1./1.0e+2)+q_dot4.*t5.*t6.*t7.*(3.9e+1./1.0e+2),q_dot4.*t3.*t5.*(-3.9e+1./1.0e+2)+q_dot2.*t7.*t9.*(3.9e+1./1.0e+2)+q_dot2.*t3.*t4.*t5.*(3.9e+1./1.0e+2)-q_dot3.*t5.*t7.*t8.*(3.9e+1./1.0e+2)-q_dot4.*t4.*t7.*t9.*(3.9e+1./1.0e+2),0.0,0.0,0.0,0.0,0.0,0.0,0.0,0.0,0.0];
j_dot = reshape([mt1,mt2,mt3,mt4],3,7);
end
